simulink model "Spring_Damper_System"  (R2021b)
settings: Solver=VariableStepAuto  StartTime=0.0  StopTime=10.0  RelTol=1e-3
settings Model: Creator=amr_y  LastModifiedBy=amr_y

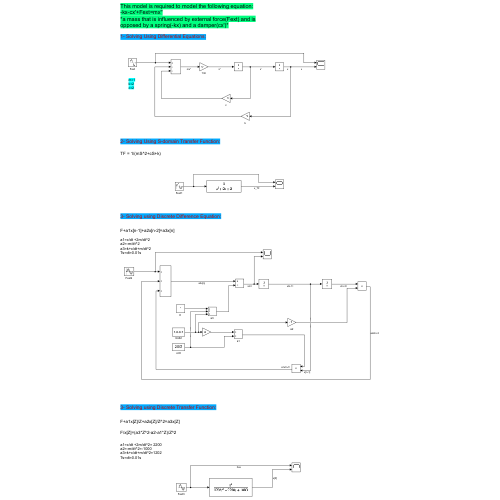
[thumbnail: Simulink's stored preview of the top-level diagram]
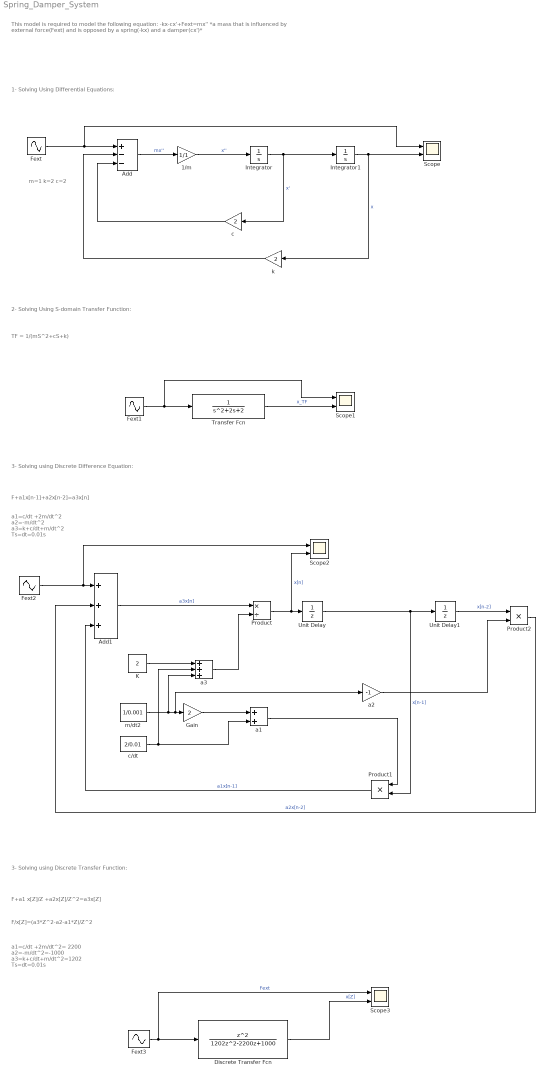
== system Spring_Damper_System ==
  note: a1=c/dt +2m/dt^2
      | a2=-m/dt^2
      | a3=k+c/dt+m/dt^2
      | Ts=dt=0.01s
  note: TF = 1/(mS^2+cS+k)
  note: 1- Solving Using Differential Equations:
  note: m=1
      | k=2
      | c=2
  note: This model is required to model the following equation:
      | -kx-cx'+Fext=mx''
      | *a mass that is influenced by external force(Fext) and is opposed by a spring(-kx) and a damper(cx')*
  note: 2- Solving Using S-domain Transfer Function:
  note: 3- Solving using Discrete Difference Equation:
  note: F+a1x[n-1]+a2x[n-2]=a3x[n]
  note: a1=c/dt +2m/dt^2= 2200
      | a2=-m/dt^2=-1000
      | a3=k+c/dt+m/dt^2=1202
      | Ts=dt=0.01s
  note: 3- Solving using Discrete Transfer Function:
  note: F+a1 x[Z]/Z +a2x[Z]/Z^2=a3x[Z]
  note: F/x[Z]=(a3*Z^2-a2-a1*Z)/Z^2
  1/m : Gain  Gain=1/1
  Add : Sum  Inputs=+--
  Add1 : Sum  Inputs=+++
  Discrete Transfer Fcn : DiscreteTransferFcn  Numerator=[1 0 0]  Denominator=[1202 -2200 1000]
  Fext : Sin  SampleTime=0
  Fext1 : Sin  SampleTime=0
  Fext2 : Sin  SampleTime=0.01
  Fext3 : Sin  SampleTime=0.01
  Gain : Gain  Gain=2
  Integrator : Integrator
  Integrator1 : Integrator
  K : Constant  Value=2
  Product : Product  Inputs=*/
  Product1 : Product
  Product2 : Product
  Scope{,1..3} (4 alike) : Scope  NumInputPorts=2
  Transfer Fcn : TransferFcn  Denominator=[1 2 2]
  Unit Delay : UnitDelay  SampleTime=-1  HasFrameUpgradeWarning=on
  Unit Delay1 : UnitDelay  SampleTime=-1  HasFrameUpgradeWarning=on
  a1 : Sum
  a2 : Gain  Gain=-1
  a3 : Sum  Inputs=+++
  c : Gain  Gain=2
  c/dt : Constant  Value=2/0.01
  k : Gain  Gain=2
  m/dt2 : Constant  Value=1/0.001
  wires:
  Integrator/1 -> c/1, Integrator1/1  "x'"
  Add/1 -> 1/m/1  "mx''"
  1/m/1 -> Integrator/1  "x''"
  Integrator1/1 -> k/1, Scope/2  "x"
  k/1 -> Add/2
  c/1 -> Add/3
  Fext/1 -> Scope/1, Add/1
  Fext1/1 -> Scope1/1, Transfer Fcn/1
  Transfer Fcn/1 -> Scope1/2  "x_TF"
  Fext2/1 -> Scope2/1, Add1/1
  Add1/1 -> Product/1  "a3x[n]"
  Unit Delay1/1 -> Product2/1  "x[n-2]"
  Product/1 -> Scope2/2, Unit Delay/1  "x[n]"
  c/dt/1 -> a3/2, a1/2
  m/dt2/1 -> a3/3, a2/1, Gain/1
  Gain/1 -> a1/1
  K/1 -> a3/1
  Unit Delay/1 -> Product1/2, Unit Delay1/1  "x[n-1]"
  a1/1 -> Product1/1
  a2/1 -> Product2/2
  Product2/1 -> Add1/2  "a2x[n-2]"
  a3/1 -> Product/2
  Product1/1 -> Add1/3  "a1x[n-1]"
  Fext3/1 -> Scope3/1, Discrete Transfer Fcn/1  "Fext"
  Discrete Transfer Fcn/1 -> Scope3/2  "x[Z]"
